simulink model "practice1"  (R2023b)
settings: Solver=VariableStepAuto  StartTime=0.0  StopTime=10.0  RelTol=1e-3
values from neighbouring files (symbols this model uses):
  a = 10    [abc.m]    (also in example1.mat; practice1_constant_val.m = 1)
  b = 13    [abc.m]    (also in example1.mat; practice1_constant_val.m = 2)
  c = a+b    (= 23)    [abc.m]    (also in example1.mat; practice1_constant_val.m = 3)
  f = input("enter the model file name")    [model_simulateautomate.m]    (also in practice1_constant_val.m = 2)
  g = 2    [practice1_constant_val.m]
  k = 2    [practice1_constant_val.m]
settings Model: Creator=39216  LastModifiedBy=39216

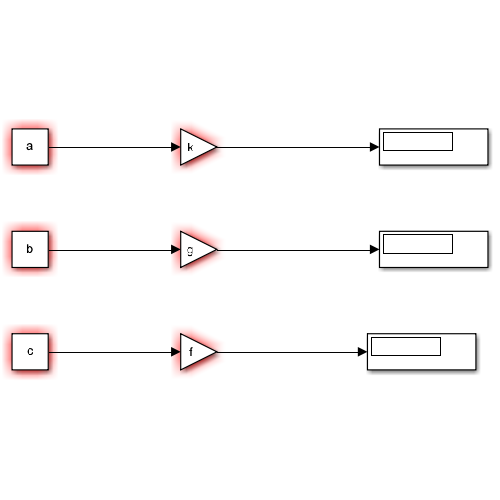
[thumbnail: Simulink's stored preview of the top-level diagram]
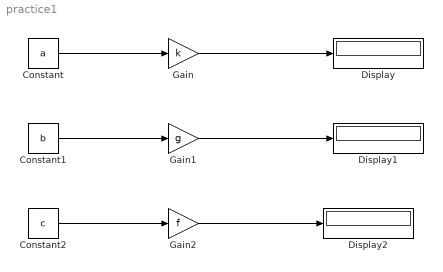
== system practice1 ==
  Constant : Constant  Value=a
  Constant1 : Constant  Value=b
  Constant2 : Constant  Value=c
  Display : Display
  Display1 : Display
  Display2 : Display
  Gain : Gain  Gain=k
  Gain1 : Gain  Gain=g
  Gain2 : Gain  Gain=f
  wires:
  Constant2/1 -> Gain2/1
  Constant1/1 -> Gain1/1
  Constant/1 -> Gain/1
  Gain/1 -> Display/1
  Gain2/1 -> Display2/1
  Gain1/1 -> Display1/1
